simulink library "lib_exhaust"  (Simulink 4.00)
undefined symbols (not defined in the file or in its folder): amb_tmp, cyc_mph, ex_cat_co_frac, ex_cat_ext_cp, ex_cat_ext_emisv, ex_cat_ext_init_tmp, ex_cat_ext_mass, ex_cat_ext_sarea, ex_cat_hc_frac, ex_cat_i2p_th_cond, ex_cat_i2x_emisv, ex_cat_i2x_th_cond, ex_cat_int_cp, ex_cat_int_init_tmp, ex_cat_int_mass, ex_cat_int_sarea, ex_cat_lim, ex_cat_m2i_th_cond, ex_cat_m2i_tmp, ex_cat_m2p_emisv, ex_cat_mon_cp, ex_cat_mon_init_tmp, ex_cat_mon_mass, ex_cat_mon_sarea, ex_cat_monf_sarea, ex_cat_moni_sarea, ex_cat_nox_frac, ex_cat_p2x_th_cond, ex_cat_pcm_ecp, ex_cat_pcm_mass, ex_cat_pcm_tmp, ex_cat_pipe_cp, ex_cat_pipe_emisv, ex_cat_pipe_init_tmp, ex_cat_pipe_mass, ex_cat_pipe_sarea, ex_cat_pm_frac, ex_cat_tmp_range, ex_gas_cp, ex_manif_cp, ex_manif_emisv, ex_manif_init_tmp, ex_manif_mass, ex_manif_sarea, ex_ornl_bool, fc_pwr_scale, magnitude
settings Model: LastModifiedBy=mokeefe
settings Model: ModifiedComment=|
  | mokeefe -- Thu Apr 18 08:32:39 2002 -- Version 1.56
  | saving the model:
  | o "without the model browser open"
  | o with only top-level screen visible
  | o with "fit to view" enabled
  | o with "status bar" off and "toolbar" off
  | o with "prompt to update model history with each save" on
settings Model: ModifiedHistory=|
  | mokeefe -- Thu Apr 18 08:32:39 2002 -- Version 1.56
  | saving the model:
  | o "without the model browser open"
  | o with only top-level screen visible
  | o with "fit to view" enabled
  | o with "status bar" off and "toolbar" off
  | o with "prompt to update model history with each save" on

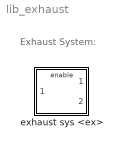
== system lib_exhaust ==
  note: Exhaust System:
  exhaust sys <ex> : Subsystem  TreatAsAtomicUnit=on
      settings: RTWFcnNameOpts=Auto  RTWFileNameOpts=Auto
      mask Display: image(imread('bdi_ex.jpg'))

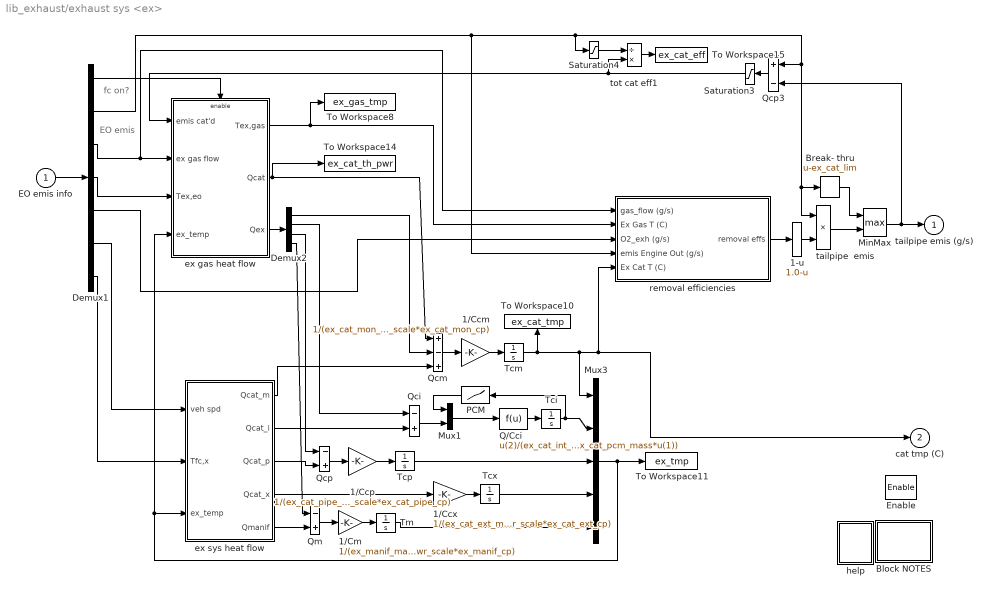
== system lib_exhaust/exhaust sys <ex> ==
  note: fc on?
  note: EO emis
  EO emis info : Inport  Port=1  LatchInput=off
  Enable : EnablePort  StatesWhenEnabling=reset
  1-u : MATLABFcn  MATLABFcn=1.0-u  OutputDimensions=-1  OutputSignalType=auto  Output1D=on
  1/Ccm : Gain  Gain=1/(ex_cat_mon_mass*fc_pwr_scale*ex_cat_mon_cp)  Multiplication=Element-wise(K.*u)  SaturateOnIntegerOverflow=on
  1/Ccp : Gain  Gain=1/(ex_cat_pipe_mass*fc_pwr_scale*ex_cat_pipe_cp)  Multiplication=Element-wise(K.*u)  SaturateOnIntegerOverflow=on
  1/Ccx : Gain  Gain=1/(ex_cat_ext_mass*fc_pwr_scale*ex_cat_ext_cp)  Multiplication=Element-wise(K.*u)  SaturateOnIntegerOverflow=on
  1/Cm : Gain  Gain=1/(ex_manif_mass*fc_pwr_scale*ex_manif_cp)  Multiplication=Element-wise(K.*u)  SaturateOnIntegerOverflow=on
  Block NOTES : Subsystem
      settings: RTWFcnNameOpts=Auto  RTWFileNameOpts=Auto
      mask Display: disp('Block\nNOTES')
  Break- thru : MATLABFcn  MATLABFcn=u-ex_cat_lim  OutputDimensions=-1  OutputSignalType=auto  Output1D=on
  Demux1 : Demux  Outputs=[1 4 1 1 1 1 4]  BusSelectionMode=off
  Demux2 : Demux  Outputs=4  BusSelectionMode=off
  MinMax : MinMax  Function=max  Inputs=2
  Mux1 : Mux  Inputs=2
      settings: DisplayOption=none
  Mux3 : Mux  Inputs=5
      settings: DisplayOption=none
  PCM : Lookup  Orientation=left  InputValues=ex_cat_pcm_tmp  OutputValues=ex_cat_pcm_ecp
  Q/Cci : Fcn  Expr=u(2)/(ex_cat_int_mass*fc_pwr_scale*ex_cat_int_cp+ex_cat_pcm_mass*u(1))
  Qci : Sum  Inputs=-+  SaturateOnIntegerOverflow=on
  Qcm : Sum  Inputs=+-+  SaturateOnIntegerOverflow=on
  Qcp : Sum  Inputs=-+  SaturateOnIntegerOverflow=on
  Qcp3 : Sum  Orientation=left  Inputs=+-  SaturateOnIntegerOverflow=on
  Qm : Sum  Inputs=-+  SaturateOnIntegerOverflow=on
  Saturation3 : Saturate  Orientation=left  UpperLimit=Inf  LowerLimit=0  LinearizeAsGain=on
  Saturation4 : Saturate  UpperLimit=Inf  LowerLimit=eps  LinearizeAsGain=on
  Tci : Integrator  ExternalReset=none  InitialConditionSource=internal  InitialCondition=ex_cat_int_init_tmp  LimitOutput=off  UpperSaturationLimit=inf  LowerSaturationLimit=-inf  ShowSaturationPort=off  ShowStatePort=off  AbsoluteTolerance=auto
  Tcm : Integrator  ExternalReset=none  InitialConditionSource=internal  InitialCondition=ex_cat_mon_init_tmp  LimitOutput=off  UpperSaturationLimit=inf  LowerSaturationLimit=-inf  ShowSaturationPort=off  ShowStatePort=off  AbsoluteTolerance=auto
  Tcp : Integrator  ExternalReset=none  InitialConditionSource=internal  InitialCondition=ex_cat_pipe_init_tmp  LimitOutput=off  UpperSaturationLimit=inf  LowerSaturationLimit=-inf  ShowSaturationPort=off  ShowStatePort=off  AbsoluteTolerance=auto
  Tcx : Integrator  ExternalReset=none  InitialConditionSource=internal  InitialCondition=ex_cat_ext_init_tmp  LimitOutput=off  UpperSaturationLimit=inf  LowerSaturationLimit=-inf  ShowSaturationPort=off  ShowStatePort=off  AbsoluteTolerance=auto
  Tm : Integrator  ExternalReset=none  InitialConditionSource=internal  InitialCondition=ex_manif_init_tmp  LimitOutput=off  UpperSaturationLimit=inf  LowerSaturationLimit=-inf  ShowSaturationPort=off  ShowStatePort=off  AbsoluteTolerance=auto
  To Workspace10 : ToWorkspace  VariableName=ex_cat_tmp  SampleTime=-1  SaveFormat=Array
      settings: Orientation=up
  To Workspace11 : ToWorkspace  VariableName=ex_tmp  SampleTime=-1  SaveFormat=Array
  To Workspace14 : ToWorkspace  VariableName=ex_cat_th_pwr  SampleTime=-1  SaveFormat=Array
  To Workspace15 : ToWorkspace  VariableName=ex_cat_eff  SampleTime=-1  SaveFormat=Array
  To Workspace8 : ToWorkspace  VariableName=ex_gas_tmp  SampleTime=-1  SaveFormat=Array
  ex gas heat flow : Subsystem  TreatAsAtomicUnit=on
      settings: RTWFcnNameOpts=Auto  RTWFileNameOpts=Auto
  ex sys heat flow : Subsystem
      settings: RTWFcnNameOpts=Auto  RTWFileNameOpts=Auto
  help : Subsystem
      settings: OpenFcn=web(['file:\\\' which('exhaust.htm')]);  RTWFcnNameOpts=Auto  RTWFileNameOpts=Auto
      mask Display: image(imread('doc_man.jpg'))
  removal efficiencies : Subsystem
      settings: RTWFcnNameOpts=Auto  RTWFileNameOpts=Auto
  tailpipe  emis : Product  Inputs=2  Multiplication=Element-wise(.*)  SaturateOnIntegerOverflow=on
  tot cat eff1 : Product  Inputs=/*  Multiplication=Element-wise(.*)  SaturateOnIntegerOverflow=on
  tailpipe emis (g/s) : Outport  Port=1  OutputWhenDisabled=reset  InitialOutput=0
  cat tmp (C) : Outport  Port=2  OutputWhenDisabled=reset  InitialOutput=0
  wires:
  ex gas heat flow/3(Qex) -> Demux2/1
  Demux1/4 -> ex gas heat flow/3(Tex,eo)
  Demux1/1 -> ex gas heat flow/Enable
  1/Ccm/1 -> Tcm/1
  Qcm/1 -> 1/Ccm/1
  ex sys heat flow/1(Qcat_m) -> Qcm/3
  Demux2/1 -> Qcm/2
  ex sys heat flow/4(Qcat_x) -> 1/Ccx/1
  ex sys heat flow/5(Qmanif) -> Qm/2
  ex sys heat flow/2(Qcat_i) -> Qci/2
  1/Ccx/1 -> Tcx/1
  1/Cm/1 -> Tm/1
  Qm/1 -> 1/Cm/1
  Q/Cci/1 -> Tci/1
  Mux1/1 -> Q/Cci/1
  PCM/1 -> Mux1/1
  Qci/1 -> Mux1/2
  Tci/1 -> PCM/1, Mux3/2
  ex sys heat flow/3(Qcat_p) -> Qcp/2
  Demux2/2 -> Qci/1
  Demux2/4 -> Qm/1
  Demux2/3 -> Qcp/1
  Tcx/1 -> Mux3/4
  Tcp/1 -> Mux3/3
  Tm/1 -> Mux3/5
  Mux3/1 -> To Workspace11/1, ex gas heat flow/4(ex_temp), ex sys heat flow/3(ex_temp)
  Tcm/1 -> Mux3/1, cat tmp (C)/1, removal efficiencies/5(Ex Cat T (C)), To Workspace10/1
  Qcp/1 -> 1/Ccp/1
  1/Ccp/1 -> Tcp/1
  ex gas heat flow/2(Qcat) -> Qcm/1, To Workspace14/1
  Break- thru/1 -> MinMax/1
  tailpipe  emis/1 -> MinMax/2
  1-u/1 -> tailpipe  emis/2
  MinMax/1 -> tailpipe emis (g/s)/1, Qcp3/2
  removal efficiencies/1(removal effs) -> 1-u/1
  Qcp3/1 -> Saturation3/1
  Saturation3/1 -> ex gas heat flow/1(emis cat'd), tot cat eff1/2
  Saturation4/1 -> tot cat eff1/1
  tot cat eff1/1 -> To Workspace15/1
  EO emis info/1 -> Demux1/1
  ex gas heat flow/1(Tex,gas) -> To Workspace8/1, removal efficiencies/2(Ex Gas T (C))
  Demux1/3 -> ex gas heat flow/2(ex gas flow), removal efficiencies/1(gas_flow (g/s))
  Demux1/2 -> Saturation4/1, tailpipe  emis/1, Break- thru/1, Qcp3/1, removal efficiencies/4(emis Engine Out (g/s))
  Demux1/6 -> ex sys heat flow/1(veh spd)
  Demux1/7 -> ex sys heat flow/2(Tfc,x)
  Demux1/5 -> removal efficiencies/3(O2_exh (g/s))

== system lib_exhaust/exhaust sys <ex>/Block NOTES ==
  note: This block models the exhaust system of an internal combustion engine (ICE).  Emphasis is on the catalytic converter
      | aftertreatment of emissions.  Since converter performance is tied to operating temperature, the temperature and heat
      | flows of the exhaust gas, converter, and engine manifold/downpipe are predicted.

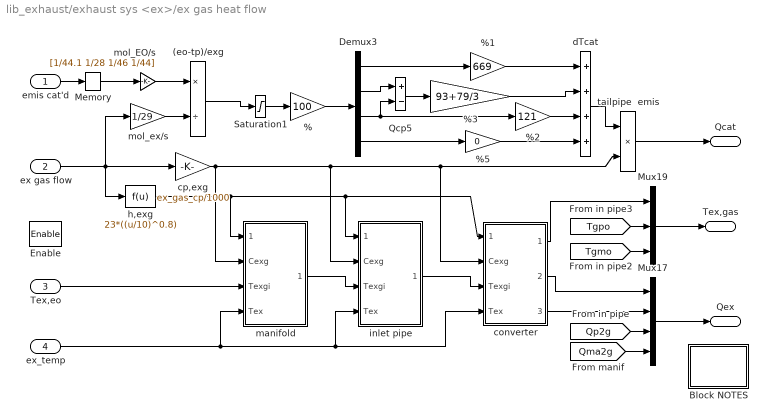
== system lib_exhaust/exhaust sys <ex>/ex gas heat flow ==
  emis cat'd : Inport  Port=1  LatchInput=off
  ex gas flow : Inport  Port=2  LatchInput=off
  Tex,eo : Inport  Port=3  LatchInput=off
  ex_temp : Inport  Port=4  LatchInput=off
  Enable : EnablePort  StatesWhenEnabling=reset
  % : Gain  Gain=100  Multiplication=Element-wise(K.*u)  SaturateOnIntegerOverflow=on
  %1 : Gain  Gain=669  Multiplication=Element-wise(K.*u)  SaturateOnIntegerOverflow=on
  %2 : Gain  Gain=121  Multiplication=Element-wise(K.*u)  SaturateOnIntegerOverflow=on
  %3 : Gain  Gain=93+79/3  Multiplication=Element-wise(K.*u)  SaturateOnIntegerOverflow=on
  %5 : Gain  Gain=0  Multiplication=Element-wise(K.*u)  SaturateOnIntegerOverflow=on
  (eo-tp)/exg : Product  Inputs=*/  Multiplication=Element-wise(.*)  SaturateOnIntegerOverflow=on
  Block NOTES : Subsystem
      settings: RTWFcnNameOpts=Auto  RTWFileNameOpts=Auto
      mask Display: disp('Block\nNOTES')
  Demux3 : Demux  Outputs=4  BusSelectionMode=off
  Memory : Memory  X0=[0 0 0 0]  InheritSampleTime=off
      settings: RTWStateStorageClass=Auto
  Mux17 : Mux  Inputs=4
      settings: DisplayOption=none
  Mux19 : Mux  Inputs=3
      settings: DisplayOption=none
  Qcp5 : Sum  Inputs=+-  SaturateOnIntegerOverflow=on
  Saturation1 : Saturate  UpperLimit=1  LowerLimit=0  LinearizeAsGain=on
  converter : Subsystem
      settings: RTWFcnNameOpts=Auto  RTWFileNameOpts=Auto
  cp,exg : Gain  Gain=ex_gas_cp/1000  Multiplication=Element-wise(K.*u)  SaturateOnIntegerOverflow=on
  dTcat : Sum  Inputs=++++  SaturateOnIntegerOverflow=on
  h,exg : Fcn  Expr=23*((u/10)^0.8)
  inlet pipe : Subsystem
      settings: RTWFcnNameOpts=Auto  RTWFileNameOpts=Auto
  "manifold " : Subsystem
      settings: RTWFcnNameOpts=Auto  RTWFileNameOpts=Auto
  mol_EO/s : Gain  Gain=[1/44.1 1/28 1/46 1/44]  Multiplication=Element-wise(K.*u)  SaturateOnIntegerOverflow=on
  mol_ex/s : Gain  Gain=1/29  Multiplication=Element-wise(K.*u)  SaturateOnIntegerOverflow=on
  tailpipe  emis : Product  Inputs=2  Multiplication=Element-wise(.*)  SaturateOnIntegerOverflow=on
  Tex,gas : Outport  Port=1  OutputWhenDisabled=reset  InitialOutput=amb_tmp
  Qcat : Outport  Port=2  OutputWhenDisabled=reset  InitialOutput=0
  Qex : Outport  Port=3  OutputWhenDisabled=reset  InitialOutput=0
  wires:
  %/1 -> Demux3/1
  h,exg/1 -> "manifold "/1(h,exg), converter/1(h,exg), inlet pipe/1(h,exg)
  cp,exg/1 -> "manifold "/2(Cexg), converter/2(Cexg), tailpipe  emis/2, inlet pipe/2(Cexg)
  ex_temp/1 -> "manifold "/4(Tex), converter/4(Tex), inlet pipe/4(Tex)
  Tex,eo/1 -> "manifold "/3(Texgi)
  (eo-tp)/exg/1 -> Saturation1/1
  mol_EO/s/1 -> (eo-tp)/exg/1
  mol_ex/s/1 -> (eo-tp)/exg/2
  Saturation1/1 -> %/1
  Demux3/4 -> %5/1
  Qcp5/1 -> %3/1
  Demux3/1 -> %1/1
  Demux3/3 -> %2/1, Qcp5/2
  Demux3/2 -> Qcp5/1
  inlet pipe/1(Texgo) -> converter/3(Texgi)
  %5/1 -> dTcat/4
  [Qma2g] -> Mux17/4
  [Qp2g] -> Mux17/3
  converter/3(Qci2g) -> Mux17/2
  converter/2(Qcm2g) -> Mux17/1
  converter/1(Texgo) -> Mux19/1
  [Tgpo] -> Mux19/2
  [Tgmo] -> Mux19/3
  Mux17/1 -> Qex/1
  Mux19/1 -> Tex,gas/1
  tailpipe  emis/1 -> Qcat/1
  dTcat/1 -> tailpipe  emis/1
  %1/1 -> dTcat/1
  %3/1 -> dTcat/2
  %2/1 -> dTcat/3
  "manifold "/1(Texgo) -> inlet pipe/3(Texgi)
  ex gas flow/1 -> mol_ex/s/1, h,exg/1, cp,exg/1
  emis cat'd/1 -> Memory/1
  Memory/1 -> mol_EO/s/1

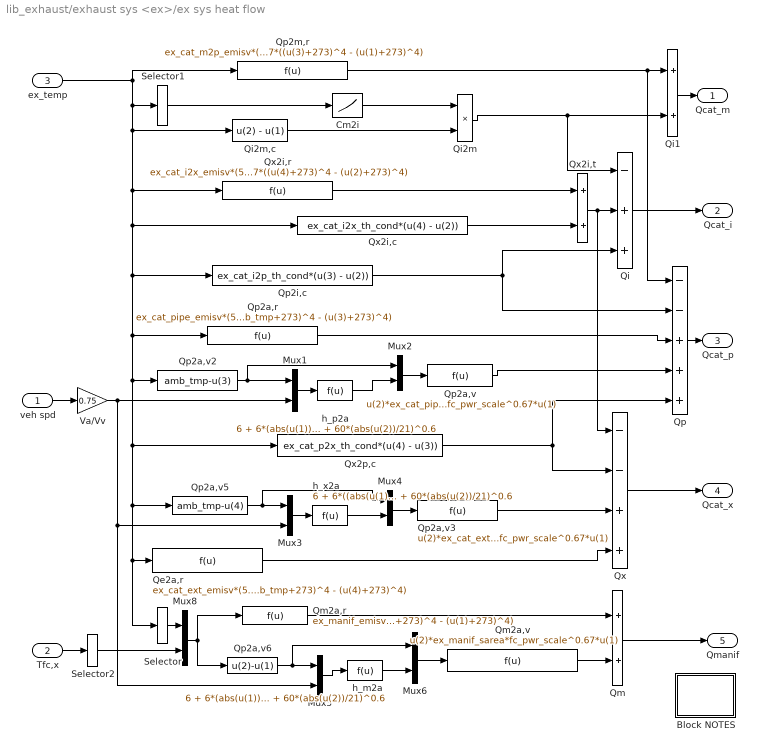
== system lib_exhaust/exhaust sys <ex>/ex sys heat flow ==
  veh spd : Inport  Port=1  LatchInput=off
  Tfc,x : Inport  Port=2  LatchInput=off
  ex_temp : Inport  Port=3  LatchInput=off
  Block NOTES : Subsystem
      settings: RTWFcnNameOpts=Auto  RTWFileNameOpts=Auto
      mask Display: disp('Block\nNOTES')
  Cm2i : Lookup  InputValues=ex_cat_m2i_tmp  OutputValues=ex_cat_m2i_th_cond
  Mux{1..6,8} (7 alike) : Mux  Inputs=2
      settings: DisplayOption=none
  Qe2a,r : Fcn  Expr=ex_cat_ext_emisv*(5.67e-8)*ex_cat_ext_sarea*fc_pwr_scale^0.67*((amb_tmp+273)^4 - (u(4)+273)^4)
  Qi : Sum  Inputs=-++  SaturateOnIntegerOverflow=on
  Qi1 : Sum  Inputs=++  SaturateOnIntegerOverflow=on
  Qi2m : Product  Inputs=2  Multiplication=Element-wise(.*)  SaturateOnIntegerOverflow=on
  Qi2m,c : Fcn  Expr=u(2) - u(1)
  Qm : Sum  Inputs=++  SaturateOnIntegerOverflow=on
  Qm2a,r : Fcn  Expr=ex_manif_emisv*(5.67e-8)*ex_manif_sarea*fc_pwr_scale^0.67*((u(2)+273)^4 - (u(1)+273)^4)
  Qm2a,v : Fcn  Expr=u(2)*ex_manif_sarea*fc_pwr_scale^0.67*u(1)
  Qp : Sum  Inputs=--+++  SaturateOnIntegerOverflow=on
  Qp2a,r : Fcn  Expr=ex_cat_pipe_emisv*(5.67e-8)*ex_cat_pipe_sarea*fc_pwr_scale^0.67*((amb_tmp+273)^4 - (u(3)+273)^4)
  Qp2a,v : Fcn  Expr=u(2)*ex_cat_pipe_sarea*fc_pwr_scale^0.67*u(1)
  Qp2a,v2 : Fcn  Expr=amb_tmp-u(3)
  Qp2a,v3 : Fcn  Expr=u(2)*ex_cat_ext_sarea*fc_pwr_scale^0.67*u(1)
  Qp2a,v5 : Fcn  Expr=amb_tmp-u(4)
  Qp2a,v6 : Fcn  Expr=u(2)-u(1)
  Qp2i,c : Fcn  Expr=ex_cat_i2p_th_cond*(u(3) - u(2))
  Qp2m,r : Fcn  Expr=ex_cat_m2p_emisv*(5.67e-8)*ex_cat_monf_sarea*fc_pwr_scale^0.67*((u(3)+273)^4 - (u(1)+273)^4)
  Qx : Sum  Inputs=--++  SaturateOnIntegerOverflow=on
  Qx2i,c : Fcn  Expr=ex_cat_i2x_th_cond*(u(4) - u(2))
  Qx2i,r : Fcn  Expr=ex_cat_i2x_emisv*(5.67e-8)*ex_cat_int_sarea*fc_pwr_scale^0.67*((u(4)+273)^4 - (u(2)+273)^4)
  Qx2i,t : Sum  Inputs=++  SaturateOnIntegerOverflow=on
  Qx2p,c : Fcn  Expr=ex_cat_p2x_th_cond*(u(4) - u(3))
  Selector : Selector  InputType=Vector  ElementSrc=Internal  Elements=5  RowSrc=Internal  Rows=1  ColumnSrc=Internal  Columns=1  InputPortWidth=5
  Selector1 : Selector  InputType=Vector  ElementSrc=Internal  Elements=[2]  RowSrc=Internal  Rows=1  ColumnSrc=Internal  Columns=1  InputPortWidth=5
  Selector2 : Selector  InputType=Vector  ElementSrc=Internal  Elements=3  RowSrc=Internal  Rows=1  ColumnSrc=Internal  Columns=1  InputPortWidth=4
  Va/Vv : Gain  Gain=0.75  Multiplication=Element-wise(K.*u)  SaturateOnIntegerOverflow=on
  h_m2a : Fcn  Expr=6 + 6*(abs(u(1))/1000)^0.3 + 60*(abs(u(2))/21)^0.6
  h_p2a : Fcn  Expr=6 + 6*(abs(u(1))/1000)^0.3 + 60*(abs(u(2))/21)^0.6
  h_x2a : Fcn  Expr=6 + 6*((abs(u(1))/1000))^0.3 + 60*(abs(u(2))/21)^0.6
  Qcat_m : Outport  Port=1
  Qcat_i : Outport  Port=2
  Qcat_p : Outport  Port=3
  Qcat_x : Outport  Port=4
  Qmanif : Outport  Port=5
  wires:
  Va/Vv/1 -> Mux1/2, Mux5/2, Mux3/2
  veh spd/1 -> Va/Vv/1
  Selector2/1 -> Mux8/2
  Tfc,x/1 -> Selector2/1
  h_m2a/1 -> Mux6/2
  Mux8/1 -> Qp2a,v6/1, Qm2a,r/1
  Selector/1 -> Mux8/1
  Qp2a,v6/1 -> Mux6/1, Mux5/1
  Mux5/1 -> h_m2a/1
  Mux6/1 -> Qm2a,v/1
  Qm2a,r/1 -> Qm/1
  Qm/1 -> Qmanif/1
  Qm2a,v/1 -> Qm/2
  Qx2p,c/1 -> Qx/2, Qp/5
  h_p2a/1 -> Mux2/2
  Mux2/1 -> Qp2a,v/1
  Qe2a,r/1 -> Qx/4
  h_x2a/1 -> Mux4/2
  Qp2a,v5/1 -> Mux4/1, Mux3/1
  Mux3/1 -> h_x2a/1
  Qp2a,v3/1 -> Qx/3
  Qx2i,t/1 -> Qx/1, Qi/2
  Qx2i,r/1 -> Qx2i,t/1
  Qp2a,v/1 -> Qp/4
  Qp2a,r/1 -> Qp/3
  Qp2m,r/1 -> Qp/1, Qi1/1
  Qp2i,c/1 -> Qp/2, Qi/3
  Cm2i/1 -> Qi2m/1
  Selector1/1 -> Cm2i/1
  Qi2m/1 -> Qi/1, Qi1/2
  Qi2m,c/1 -> Qi2m/2
  Qx2i,c/1 -> Qx2i,t/2
  Qi1/1 -> Qcat_m/1
  Qx/1 -> Qcat_x/1
  Mux4/1 -> Qp2a,v3/1
  Qp2a,v2/1 -> Mux2/1, Mux1/1
  Mux1/1 -> h_p2a/1
  Qp/1 -> Qcat_p/1
  Qi/1 -> Qcat_i/1
  ex_temp/1 -> Selector/1, Qe2a,r/1, Qp2a,v5/1, Qx2p,c/1, Qp2a,v2/1, Qp2a,r/1, Qp2i,c/1, Qi2m,c/1, Selector1/1, Qp2m,r/1, Qx2i,r/1, Qx2i,c/1

== system lib_exhaust/exhaust sys <ex>/help ==

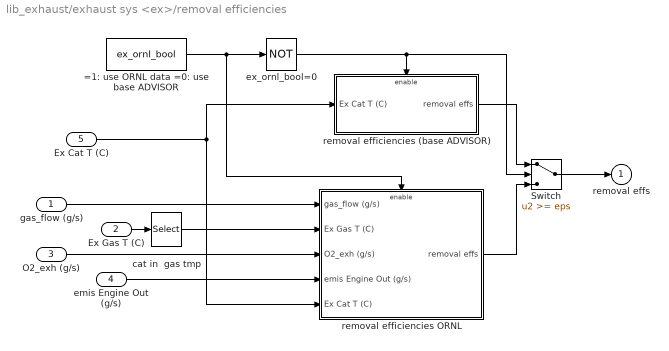
== system lib_exhaust/exhaust sys <ex>/removal efficiencies ==
  gas_flow (g/s) : Inport  Port=1  LatchInput=off
  Ex Gas T (C) : Inport  Port=2  LatchInput=off
  O2_exh (g/s) : Inport  Port=3  LatchInput=off
  emis Engine Out (g/s) : Inport  Port=4  LatchInput=off
  Ex Cat T (C) : Inport  Port=5  LatchInput=off
  =1: use ORNL data =0: use base ADVISOR : Constant  Value=ex_ornl_bool
  Switch : Switch  Threshold=eps
  cat in  gas tmp : Selector  InputType=Vector  ElementSrc=Internal  Elements=2  RowSrc=Internal  Rows=1  ColumnSrc=Internal  Columns=1  InputPortWidth=3
  ex_ornl_bool=0 : Logic  Operator=NOT  Inputs=2
  removal efficiencies (base ADVISOR) : Subsystem  TreatAsAtomicUnit=on
      settings: RTWFcnNameOpts=Auto  RTWFileNameOpts=Auto
  removal efficiencies ORNL : Subsystem  TreatAsAtomicUnit=on
      settings: RTWFcnNameOpts=Auto  RTWFileNameOpts=Auto
  removal effs : Outport  Port=1  OutputWhenDisabled=reset  InitialOutput=0
  wires:
  ex_ornl_bool=0/1 -> removal efficiencies (base ADVISOR)/Enable, Switch/2
  Ex Cat T (C)/1 -> removal efficiencies (base ADVISOR)/1(Ex Cat T (C)), removal efficiencies ORNL/5(Ex Cat T (C))
  Switch/1 -> removal effs/1
  Ex Gas T (C)/1 -> cat in  gas tmp/1
  cat in  gas tmp/1 -> removal efficiencies ORNL/2(Ex Gas T (C))
  emis Engine Out (g/s)/1 -> removal efficiencies ORNL/4(emis Engine Out (g/s))
  gas_flow (g/s)/1 -> removal efficiencies ORNL/1(gas_flow (g/s))
  O2_exh (g/s)/1 -> removal efficiencies ORNL/3(O2_exh (g/s))
  =1: use ORNL data =0: use base ADVISOR/1 -> ex_ornl_bool=0/1, removal efficiencies ORNL/Enable
  removal efficiencies ORNL/1(removal effs) -> Switch/3
  removal efficiencies (base ADVISOR)/1(removal effs) -> Switch/1

== system lib_exhaust/exhaust sys <ex>/ex gas heat flow/Block NOTES ==
  note: EXHAUST GAS HEAT TRANSFER
      | This block models the heat loss from the exhaust gas as it flows from the engine through the manifold,
      | downpipe, and catalytic converter.  Also included is the increase in gas temperature within the converter
      | due to the catalysis of HC, CO, and NOx. The block is conditionally executed only if engine_on=1.

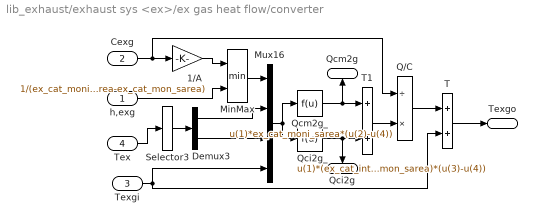
== system lib_exhaust/exhaust sys <ex>/ex gas heat flow/converter ==
  h,exg : Inport  Port=1  LatchInput=off
  Cexg : Inport  Port=2  LatchInput=off
  Texgi : Inport  Port=3  LatchInput=off
  Tex : Inport  Port=4  LatchInput=off
  " Q/C" : Product  Inputs=/*  Multiplication=Element-wise(.*)  SaturateOnIntegerOverflow=on
  1/A : Gain  Gain=1/(ex_cat_moni_sarea+ex_cat_int_sarea-ex_cat_mon_sarea)  Multiplication=Element-wise(K.*u)  SaturateOnIntegerOverflow=on
  Demux3 : Demux  Outputs=2  BusSelectionMode=off
  MinMax : MinMax  Function=min  Inputs=2
  Mux16 : Mux  Inputs=4
      settings: DisplayOption=none
  Qci2g_ : Fcn  Expr=u(1)*(ex_cat_int_sarea - ex_cat_mon_sarea)*(u(3)-u(4))
  Qcm2g_ : Fcn  Expr=u(1)*ex_cat_moni_sarea*(u(2)-u(4))
  Selector3 : Selector  InputType=Vector  ElementSrc=Internal  Elements=[ 1 2 ]  RowSrc=Internal  Rows=1  ColumnSrc=Internal  Columns=1  InputPortWidth=5
  T : Sum  Inputs=++  SaturateOnIntegerOverflow=on
  T1 : Sum  Inputs=++  SaturateOnIntegerOverflow=on
  Texgo : Outport  Port=1  OutputWhenDisabled=reset  InitialOutput=amb_tmp
  Qcm2g : Outport  Orientation=up  Port=2  OutputWhenDisabled=reset  InitialOutput=0
  Qci2g : Outport  Orientation=down  Port=3  OutputWhenDisabled=reset  InitialOutput=0
  wires:
  T/1 -> Texgo/1
  T1/1 -> " Q/C"/2
  " Q/C"/1 -> T/1
  Qcm2g_/1 -> Qcm2g/1, T1/1
  Qci2g_/1 -> Qci2g/1, T1/2
  Mux16/1 -> Qci2g_/1, Qcm2g_/1
  Texgi/1 -> Mux16/4, T/2
  Demux3/2 -> Mux16/3
  Demux3/1 -> Mux16/2
  Selector3/1 -> Demux3/1
  Tex/1 -> Selector3/1
  MinMax/1 -> Mux16/1
  1/A/1 -> MinMax/1
  h,exg/1 -> MinMax/2
  Cexg/1 -> 1/A/1, " Q/C"/1

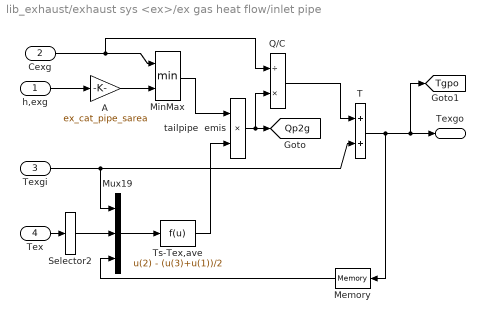
== system lib_exhaust/exhaust sys <ex>/ex gas heat flow/inlet pipe ==
  h,exg : Inport  Port=1  LatchInput=off
  Cexg : Inport  Port=2  LatchInput=off
  Texgi : Inport  Port=3  LatchInput=off
  Tex : Inport  Port=4  LatchInput=off
  " Q/C" : Product  Inputs=/*  Multiplication=Element-wise(.*)  SaturateOnIntegerOverflow=on
  A : Gain  Gain=ex_cat_pipe_sarea  Multiplication=Element-wise(K.*u)  SaturateOnIntegerOverflow=on
  Memory : Memory  Orientation=left  X0=cyc_mph(1,2)*.447  InheritSampleTime=off
      settings: RTWStateStorageClass=Auto
  MinMax : MinMax  Function=min  Inputs=2
  Mux19 : Mux  Inputs=3
      settings: DisplayOption=none
  Selector2 : Selector  InputType=Vector  ElementSrc=Internal  Elements=3  RowSrc=Internal  Rows=1  ColumnSrc=Internal  Columns=1  InputPortWidth=5
  T : Sum  Inputs=++  SaturateOnIntegerOverflow=on
  Ts-Tex,ave : Fcn  Expr=u(2) - (u(3)+u(1))/2
  tailpipe  emis : Product  Inputs=2  Multiplication=Element-wise(.*)  SaturateOnIntegerOverflow=on
  Texgo : Outport  Port=1  OutputWhenDisabled=reset  InitialOutput=amb_tmp
  tag scope: Qp2g=global, Tgpo=global
  wires:
  Memory/1 -> Mux19/3
  Selector2/1 -> Mux19/2
  Ts-Tex,ave/1 -> tailpipe  emis/2
  Mux19/1 -> Ts-Tex,ave/1
  Tex/1 -> Selector2/1
  T/1 -> Memory/1, [Tgpo], Texgo/1
  Texgi/1 -> Mux19/1, T/2
  " Q/C"/1 -> T/1
  tailpipe  emis/1 -> [Qp2g], " Q/C"/2
  Cexg/1 -> " Q/C"/1, MinMax/1
  A/1 -> MinMax/2
  MinMax/1 -> tailpipe  emis/1
  h,exg/1 -> A/1

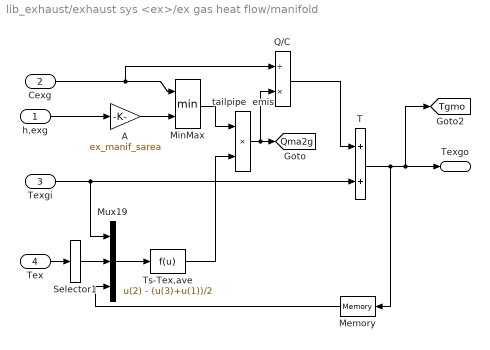
== system lib_exhaust/exhaust sys <ex>/ex gas heat flow/manifold  ==
  h,exg : Inport  Port=1  LatchInput=off
  Cexg : Inport  Port=2  LatchInput=off
  Texgi : Inport  Port=3  LatchInput=off
  Tex : Inport  Port=4  LatchInput=off
  " Q/C" : Product  Inputs=/*  Multiplication=Element-wise(.*)  SaturateOnIntegerOverflow=on
  A : Gain  Gain=ex_manif_sarea  Multiplication=Element-wise(K.*u)  SaturateOnIntegerOverflow=on
  Memory : Memory  Orientation=left  X0=cyc_mph(1,2)*.447  InheritSampleTime=off
      settings: RTWStateStorageClass=Auto
  MinMax : MinMax  Function=min  Inputs=2
  Mux19 : Mux  Inputs=3
      settings: DisplayOption=none
  Selector1 : Selector  InputType=Vector  ElementSrc=Internal  Elements=5  RowSrc=Internal  Rows=1  ColumnSrc=Internal  Columns=1  InputPortWidth=5
  T : Sum  Inputs=++  SaturateOnIntegerOverflow=on
  Ts-Tex,ave : Fcn  Expr=u(2) - (u(3)+u(1))/2
  tailpipe  emis : Product  Inputs=2  Multiplication=Element-wise(.*)  SaturateOnIntegerOverflow=on
  Texgo : Outport  Port=1  OutputWhenDisabled=reset  InitialOutput=amb_tmp
  tag scope: Qma2g=global, Tgmo=global
  wires:
  Texgi/1 -> T/2, Mux19/1
  Ts-Tex,ave/1 -> tailpipe  emis/2
  Memory/1 -> Mux19/3
  Mux19/1 -> Ts-Tex,ave/1
  Selector1/1 -> Mux19/2
  Tex/1 -> Selector1/1
  tailpipe  emis/1 -> [Qma2g], " Q/C"/2
  T/1 -> Memory/1, Texgo/1, [Tgmo]
  " Q/C"/1 -> T/1
  Cexg/1 -> " Q/C"/1, MinMax/1
  A/1 -> MinMax/2
  MinMax/1 -> tailpipe  emis/1
  h,exg/1 -> A/1

== system lib_exhaust/exhaust sys <ex>/ex sys heat flow/Block NOTES ==
  note: CATALYTIC CONVERTER HEAT LOSS
      | This block models the heat loss from a catalytic converter (conventional or vacuum-insulated).
      | Convection (as a function of vehicle speed), radiation, and conduction effects are included.
      | Converter monolith (m), interior (i), pipe (p), and exterior (x) and engine manifold
      | heat flows are estimated based on the temperatures from the previous iteration.

== system lib_exhaust/exhaust sys <ex>/removal efficiencies/removal efficiencies (base ADVISOR) ==
  Ex Cat T (C) : Inport  Port=1  LatchInput=off
  Enable : EnablePort  StatesWhenEnabling=reset
  CO temp eff : Lookup  InputValues=ex_cat_tmp_range  OutputValues=ex_cat_co_frac
  HC temp eff : Lookup  InputValues=ex_cat_tmp_range  OutputValues=ex_cat_hc_frac
  Mux : Mux  Inputs=4
      settings: DisplayOption=none
  NOx temp eff : Lookup  InputValues=ex_cat_tmp_range  OutputValues=ex_cat_nox_frac
  PM temp eff : Lookup  InputValues=ex_cat_tmp_range  OutputValues=ex_cat_pm_frac
  removal effs : Outport  Port=1  OutputWhenDisabled=reset  InitialOutput=0
  wires:
  CO temp eff/1 -> Mux/2
  HC temp eff/1 -> Mux/1
  NOx temp eff/1 -> Mux/3
  PM temp eff/1 -> Mux/4
  Mux/1 -> removal effs/1
  Ex Cat T (C)/1 -> HC temp eff/1, CO temp eff/1, NOx temp eff/1, PM temp eff/1

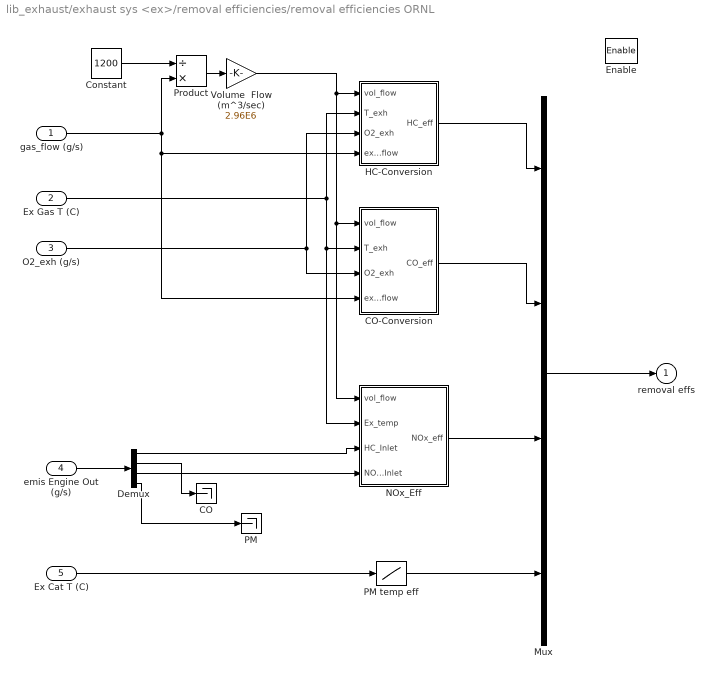
== system lib_exhaust/exhaust sys <ex>/removal efficiencies/removal efficiencies ORNL ==
  gas_flow (g/s) : Inport  Port=1  LatchInput=off
  Ex Gas T (C) : Inport  Port=2  LatchInput=off
  O2_exh (g/s) : Inport  Port=3  LatchInput=off
  emis Engine Out (g/s) : Inport  Port=4  LatchInput=off
  Ex Cat T (C) : Inport  Port=5  LatchInput=off
  Enable : EnablePort  StatesWhenEnabling=reset
  CO : Terminator
  CO-Conversion : Subsystem
      settings: RTWFcnNameOpts=Auto  RTWFileNameOpts=Auto
  Constant : Constant  Value=1200
  Demux : Demux  Outputs=4  BusSelectionMode=off
  HC-Conversion : Subsystem
      settings: RTWFcnNameOpts=Auto  RTWFileNameOpts=Auto
  Mux : Mux  Inputs=4
      settings: DisplayOption=none
  NOx_Eff : Subsystem
      settings: RTWFcnNameOpts=Auto  RTWFileNameOpts=Auto
  PM : Terminator
  PM temp eff : Lookup  InputValues=ex_cat_tmp_range  OutputValues=ex_cat_pm_frac
  Product : Product  Inputs=/*  Multiplication=Element-wise(.*)  SaturateOnIntegerOverflow=on
  Volume  Flow (m^3/sec) : Gain  Gain=2.96E6  Multiplication=Element-wise(K.*u)  SaturateOnIntegerOverflow=on
  removal effs : Outport  Port=1  OutputWhenDisabled=reset  InitialOutput=0
  wires:
  Product/1 -> Volume  Flow (m^3/sec)/1
  Constant/1 -> Product/1
  emis Engine Out (g/s)/1 -> Demux/1
  Demux/4 -> PM/1
  Demux/2 -> CO/1
  Demux/3 -> NOx_Eff/4(NOx_Inlet)
  Demux/1 -> NOx_Eff/3(HC_Inlet)
  Volume  Flow (m^3/sec)/1 -> HC-Conversion/1(vol_flow), CO-Conversion/1(vol_flow), NOx_Eff/1(vol_flow)
  Ex Gas T (C)/1 -> HC-Conversion/2(T_exh), CO-Conversion/2(T_exh), NOx_Eff/2(Ex_temp)
  PM temp eff/1 -> Mux/4
  NOx_Eff/1(NOx_eff) -> Mux/3
  HC-Conversion/1(HC_eff) -> Mux/1
  CO-Conversion/1(CO_eff) -> Mux/2
  O2_exh (g/s)/1 -> HC-Conversion/3(O2_exh), CO-Conversion/3(O2_exh)
  Ex Cat T (C)/1 -> PM temp eff/1
  gas_flow (g/s)/1 -> Product/2, HC-Conversion/4(ex_gas_flow), CO-Conversion/4(ex_gas_flow)
  Mux/1 -> removal effs/1

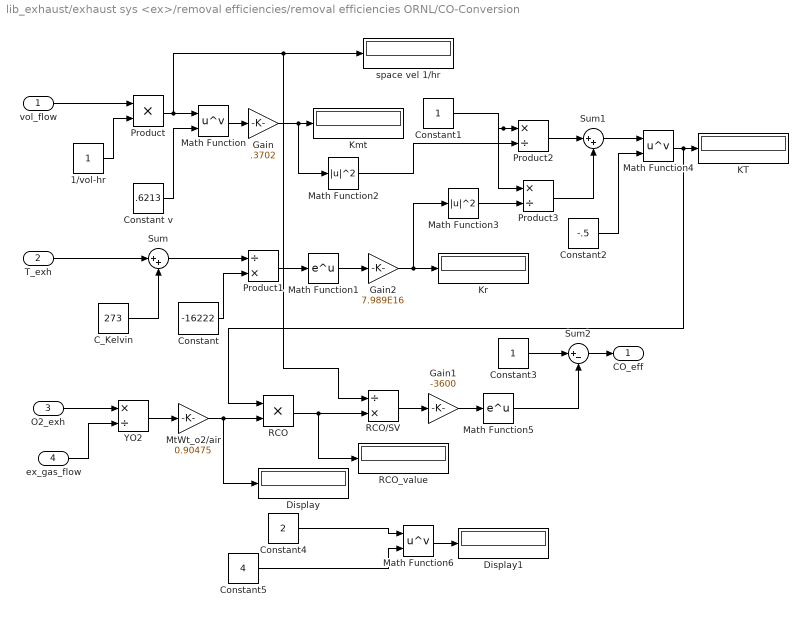
== system lib_exhaust/exhaust sys <ex>/removal efficiencies/removal efficiencies ORNL/CO-Conversion ==
  vol_flow : Inport  Port=1  LatchInput=off
  T_exh : Inport  Port=2  LatchInput=off
  O2_exh : Inport  Port=3  LatchInput=off
  ex_gas_flow : Inport  Port=4  LatchInput=off
  1/vol-hr : Constant  Value=1
  C_Kelvin : Constant  Value=273
  Constant : Constant  Value=-16222
  Constant v : Constant  Value=.6213
  Constant1 : Constant  Value=1
  Constant2 : Constant  Value=-.5
  Constant3 : Constant  Value=1
  Constant4 : Constant  Value=2
  Constant5 : Constant  Value=4
  Display : Display
      settings: Format=short
  Display1 : Display
      settings: Format=short
  Gain : Gain  Gain=.3702  Multiplication=Element-wise(K.*u)  SaturateOnIntegerOverflow=on
  Gain1 : Gain  Gain=-3600  Multiplication=Element-wise(K.*u)  SaturateOnIntegerOverflow=on
  Gain2 : Gain  Gain=7.989E16  Multiplication=Element-wise(K.*u)  SaturateOnIntegerOverflow=on
  KT : Display
      settings: Format=short_e
  Kmt : Display
      settings: Format=short_e
  Kr : Display
      settings: Format=short
  Math Function : Math  Operator=pow  OutputSignalType=auto
  Math Function1 : Math  Operator=exp  OutputSignalType=auto
  Math Function2 : Math  Operator=magnitude^2  OutputSignalType=auto
  Math Function3 : Math  Operator=magnitude^2  OutputSignalType=auto
  Math Function4 : Math  Operator=pow  OutputSignalType=auto
  Math Function5 : Math  Operator=exp  OutputSignalType=auto
  Math Function6 : Math  Operator=pow  OutputSignalType=auto
  MtWt_o2/air : Gain  Gain=0.90475  Multiplication=Element-wise(K.*u)  SaturateOnIntegerOverflow=on
  Product : Product  Inputs=2  Multiplication=Element-wise(.*)  SaturateOnIntegerOverflow=on
  Product1 : Product  Inputs=/*  Multiplication=Element-wise(.*)  SaturateOnIntegerOverflow=on
  Product2 : Product  Inputs=*/  Multiplication=Element-wise(.*)  SaturateOnIntegerOverflow=on
  Product3 : Product  Inputs=*/  Multiplication=Element-wise(.*)  SaturateOnIntegerOverflow=on
  RCO : Product  Inputs=2  Multiplication=Element-wise(.*)  SaturateOnIntegerOverflow=on
  RCO/SV : Product  Inputs=/*  Multiplication=Element-wise(.*)  SaturateOnIntegerOverflow=on
  RCO_value : Display
      settings: Format=short
  Sum : Sum  Inputs=|++  SaturateOnIntegerOverflow=on
  Sum1 : Sum  Inputs=|++  SaturateOnIntegerOverflow=on
  Sum2 : Sum  Inputs=|+-  SaturateOnIntegerOverflow=on
  YO2 : Product  Inputs=*/  Multiplication=Element-wise(.*)  SaturateOnIntegerOverflow=on
  space vel 1/hr : Display
      settings: Format=short_e
  CO_eff : Outport  Port=1
  wires:
  1/vol-hr/1 -> Product/2
  Constant v/1 -> Math Function/2
  Math Function/1 -> Gain/1
  Product/1 -> Math Function/1, space vel 1/hr/1, RCO/SV/1
  C_Kelvin/1 -> Sum/2
  Constant/1 -> Product1/2
  Sum/1 -> Product1/1
  Math Function1/1 -> Gain2/1
  Gain/1 -> Kmt/1, Math Function2/1
  Gain2/1 -> Kr/1, Math Function3/1
  Constant1/1 -> Product3/1, Product2/1
  Math Function2/1 -> Product2/2
  Math Function3/1 -> Product3/2
  Product2/1 -> Sum1/1
  Product3/1 -> Sum1/2
  Sum1/1 -> Math Function4/1
  Constant2/1 -> Math Function4/2
  Product1/1 -> Math Function1/1
  vol_flow/1 -> Product/1
  T_exh/1 -> Sum/1
  O2_exh/1 -> YO2/1
  ex_gas_flow/1 -> YO2/2
  Math Function4/1 -> KT/1, RCO/1
  RCO/SV/1 -> Gain1/1
  Gain1/1 -> Math Function5/1
  Constant3/1 -> Sum2/1
  Math Function5/1 -> Sum2/2
  Sum2/1 -> CO_eff/1
  RCO/1 -> RCO/SV/2, RCO_value/1
  YO2/1 -> MtWt_o2/air/1
  MtWt_o2/air/1 -> RCO/2, Display/1
  Constant4/1 -> Math Function6/1
  Constant5/1 -> Math Function6/2
  Math Function6/1 -> Display1/1

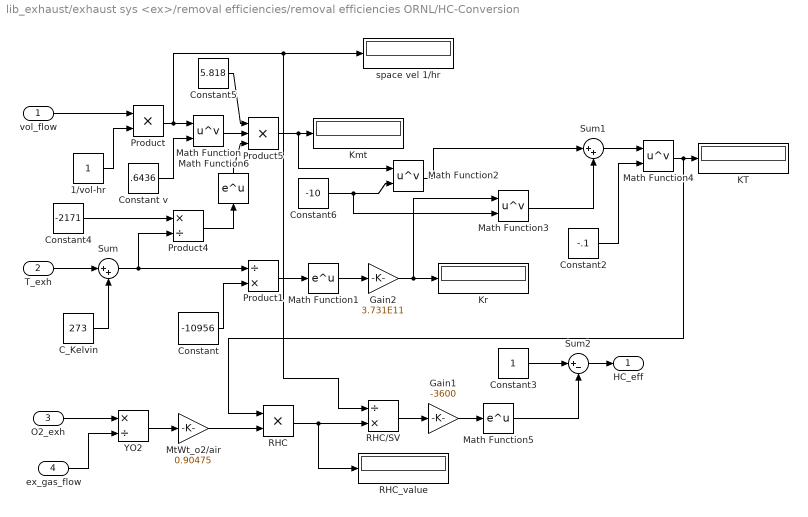
== system lib_exhaust/exhaust sys <ex>/removal efficiencies/removal efficiencies ORNL/HC-Conversion ==
  vol_flow : Inport  Port=1  LatchInput=off
  T_exh : Inport  Port=2  LatchInput=off
  O2_exh : Inport  Port=3  LatchInput=off
  ex_gas_flow : Inport  Port=4  LatchInput=off
  1/vol-hr : Constant  Value=1
  C_Kelvin : Constant  Value=273
  Constant : Constant  Value=-10956
  Constant v : Constant  Value=.6436
  Constant2 : Constant  Value=-.1
  Constant3 : Constant  Value=1
  Constant4 : Constant  Value=-2171
  Constant5 : Constant  Value=5.818
  Constant6 : Constant  Value=-10
  Gain1 : Gain  Gain=-3600  Multiplication=Element-wise(K.*u)  SaturateOnIntegerOverflow=on
  Gain2 : Gain  Gain=3.731E11  Multiplication=Element-wise(K.*u)  SaturateOnIntegerOverflow=on
  KT : Display
      settings: Format=short_e
  Kmt : Display
      settings: Format=short_e
  Kr : Display
      settings: Format=short
  Math Function{,2..4} (4 alike) : Math  Operator=pow  OutputSignalType=auto
  Math Function1 : Math  Operator=exp  OutputSignalType=auto
  Math Function5 : Math  Operator=exp  OutputSignalType=auto
  Math Function6 : Math  Orientation=up  Operator=exp  OutputSignalType=auto
  MtWt_o2/air : Gain  Gain=0.90475  Multiplication=Element-wise(K.*u)  SaturateOnIntegerOverflow=on
  Product : Product  Inputs=2  Multiplication=Element-wise(.*)  SaturateOnIntegerOverflow=on
  Product1 : Product  Inputs=/*  Multiplication=Element-wise(.*)  SaturateOnIntegerOverflow=on
  Product4 : Product  Inputs=*/  Multiplication=Element-wise(.*)  SaturateOnIntegerOverflow=on
  Product5 : Product  Inputs=3  Multiplication=Element-wise(.*)  SaturateOnIntegerOverflow=on
  RHC : Product  Inputs=2  Multiplication=Element-wise(.*)  SaturateOnIntegerOverflow=on
  RHC/SV : Product  Inputs=/*  Multiplication=Element-wise(.*)  SaturateOnIntegerOverflow=on
  RHC_value : Display
      settings: Format=short
  Sum : Sum  Inputs=|++  SaturateOnIntegerOverflow=on
  Sum1 : Sum  Inputs=|++  SaturateOnIntegerOverflow=on
  Sum2 : Sum  Inputs=|+-  SaturateOnIntegerOverflow=on
  YO2 : Product  Inputs=*/  Multiplication=Element-wise(.*)  SaturateOnIntegerOverflow=on
  space vel 1/hr : Display
      settings: Format=short_e
  HC_eff : Outport  Port=1
  wires:
  1/vol-hr/1 -> Product/2
  Constant v/1 -> Math Function/2
  Math Function/1 -> Product5/2
  Product/1 -> Math Function/1, space vel 1/hr/1, RHC/SV/1
  C_Kelvin/1 -> Sum/2
  Constant/1 -> Product1/2
  Math Function1/1 -> Gain2/1
  Product5/1 -> Kmt/1, Math Function2/1
  Gain2/1 -> Kr/1, Math Function3/1
  Sum1/1 -> Math Function4/1
  Constant2/1 -> Math Function4/2
  Product1/1 -> Math Function1/1
  vol_flow/1 -> Product/1
  O2_exh/1 -> YO2/1
  ex_gas_flow/1 -> YO2/2
  Math Function4/1 -> KT/1, RHC/1
  RHC/SV/1 -> Gain1/1
  Gain1/1 -> Math Function5/1
  Constant3/1 -> Sum2/1
  Math Function5/1 -> Sum2/2
  Sum2/1 -> HC_eff/1
  YO2/1 -> MtWt_o2/air/1
  MtWt_o2/air/1 -> RHC/2
  RHC/1 -> RHC/SV/2, RHC_value/1
  Constant4/1 -> Product4/1
  Product4/1 -> Math Function6/1
  Constant5/1 -> Product5/1
  Math Function6/1 -> Product5/3
  Constant6/1 -> Math Function2/2, Math Function3/2
  Math Function2/1 -> Sum1/1
  Math Function3/1 -> Sum1/2
  T_exh/1 -> Sum/1
  Sum/1 -> Product1/1, Product4/2

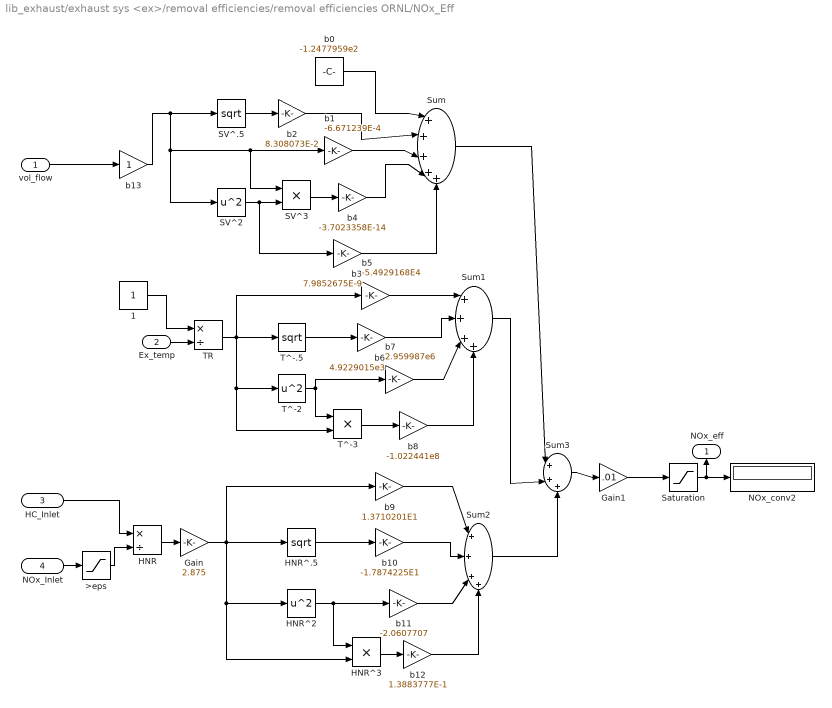
== system lib_exhaust/exhaust sys <ex>/removal efficiencies/removal efficiencies ORNL/NOx_Eff ==
  vol_flow : Inport  Port=1  LatchInput=off
  Ex_temp : Inport  Port=2  LatchInput=off
  HC_Inlet : Inport  Port=3  LatchInput=off
  NOx_Inlet : Inport  Port=4  LatchInput=off
  1 : Constant  Value=1
  >eps : Saturate  UpperLimit=inf  LowerLimit=eps  LinearizeAsGain=on
  Gain : Gain  Gain=2.875  Multiplication=Element-wise(K.*u)  SaturateOnIntegerOverflow=on
  Gain1 : Gain  Gain=.01  Multiplication=Element-wise(K.*u)  SaturateOnIntegerOverflow=on
  HNR : Product  Inputs=*/  Multiplication=Element-wise(.*)  SaturateOnIntegerOverflow=on
  HNR^.5 : Math  Operator=sqrt  OutputSignalType=auto
  HNR^2 : Math  Operator=square  OutputSignalType=auto
  HNR^3 : Product  Inputs=2  Multiplication=Element-wise(.*)  SaturateOnIntegerOverflow=on
  NOx_conv2 : Display
      settings: Format=short
  SV^.5 : Math  Operator=sqrt  OutputSignalType=auto
  SV^2 : Math  Operator=square  OutputSignalType=auto
  SV^3 : Product  Inputs=2  Multiplication=Element-wise(.*)  SaturateOnIntegerOverflow=on
  Saturation : Saturate  UpperLimit=1.0  LowerLimit=0.0  LinearizeAsGain=on
  Sum : Sum  Inputs=|+++++  SaturateOnIntegerOverflow=on
  Sum1 : Sum  Inputs=|++++  SaturateOnIntegerOverflow=on
  Sum2 : Sum  Inputs=|++++  SaturateOnIntegerOverflow=on
  Sum3 : Sum  Inputs=|+++  SaturateOnIntegerOverflow=on
  TR : Product  Inputs=*/  Multiplication=Element-wise(.*)  SaturateOnIntegerOverflow=on
  T^-.5 : Math  Operator=sqrt  OutputSignalType=auto
  T^-2 : Math  Operator=square  OutputSignalType=auto
  T^-3 : Product  Inputs=2  Multiplication=Element-wise(.*)  SaturateOnIntegerOverflow=on
  b0 : Constant  Value=-1.2477959e2
  b1 : Gain  Gain=-6.671239E-4  Multiplication=Element-wise(K.*u)  SaturateOnIntegerOverflow=on
  b10 : Gain  Gain=-1.7874225E1  Multiplication=Element-wise(K.*u)  SaturateOnIntegerOverflow=on
  b11 : Gain  Gain=-2.0607707  Multiplication=Element-wise(K.*u)  SaturateOnIntegerOverflow=on
  b12 : Gain  Gain=1.3883777E-1  Multiplication=Element-wise(K.*u)  SaturateOnIntegerOverflow=on
  b13 : Gain  Gain=1  Multiplication=Element-wise(K.*u)  SaturateOnIntegerOverflow=on
  b2 : Gain  Gain=8.308073E-2  Multiplication=Element-wise(K.*u)  SaturateOnIntegerOverflow=on
  b3 : Gain  Gain=7.9852675E-9  Multiplication=Element-wise(K.*u)  SaturateOnIntegerOverflow=on
  b4 : Gain  Gain=-3.7023358E-14  Multiplication=Element-wise(K.*u)  SaturateOnIntegerOverflow=on
  b5 : Gain  Gain=-5.4929168E4  Multiplication=Element-wise(K.*u)  SaturateOnIntegerOverflow=on
  b6 : Gain  Gain=4.9229015e3  Multiplication=Element-wise(K.*u)  SaturateOnIntegerOverflow=on
  b7 : Gain  Gain=2.959987e6  Multiplication=Element-wise(K.*u)  SaturateOnIntegerOverflow=on
  b8 : Gain  Gain=-1.022441e8  Multiplication=Element-wise(K.*u)  SaturateOnIntegerOverflow=on
  b9 : Gain  Gain=1.3710201E1  Multiplication=Element-wise(K.*u)  SaturateOnIntegerOverflow=on
  NOx_eff : Outport  Orientation=up  Port=1
  wires:
  vol_flow/1 -> b13/1
  SV^3/1 -> b4/1
  SV^2/1 -> SV^3/2, b3/1
  SV^.5/1 -> b2/1
  b0/1 -> Sum/1
  b2/1 -> Sum/2
  b1/1 -> Sum/3
  b4/1 -> Sum/4
  b3/1 -> Sum/5
  1/1 -> TR/1
  TR/1 -> T^-.5/1, T^-2/1, T^-3/2, b5/1
  T^-3/1 -> b8/1
  T^-2/1 -> T^-3/1, b7/1
  T^-.5/1 -> b6/1
  b5/1 -> Sum1/1
  b6/1 -> Sum1/2
  b7/1 -> Sum1/3
  b8/1 -> Sum1/4
  HNR^3/1 -> b12/1
  HNR^2/1 -> HNR^3/1, b11/1
  HNR^.5/1 -> b10/1
  b9/1 -> Sum2/1
  b10/1 -> Sum2/2
  b11/1 -> Sum2/3
  b12/1 -> Sum2/4
  Sum2/1 -> Sum3/3
  Sum1/1 -> Sum3/2
  Sum/1 -> Sum3/1
  HNR/1 -> Gain/1
  Gain/1 -> HNR^.5/1, b9/1, HNR^3/2, HNR^2/1
  Sum3/1 -> Gain1/1
  Gain1/1 -> Saturation/1
  b13/1 -> SV^.5/1, SV^2/1, b1/1, SV^3/1
  HC_Inlet/1 -> HNR/1
  Ex_temp/1 -> TR/2
  Saturation/1 -> NOx_conv2/1, NOx_eff/1
  NOx_Inlet/1 -> >eps/1
  >eps/1 -> HNR/2
